simulink model "backstepping"  (R2025b)
settings: Solver=VariableStepAuto  StartTime=0.0  StopTime=10.0  RelTol=1e-3
settings Model: Creator=Predrag  LastModifiedBy=Predrag

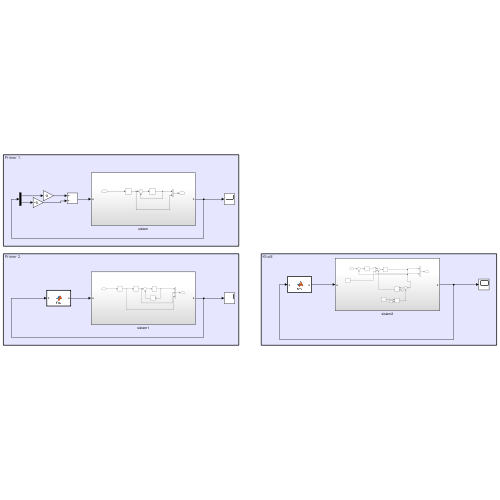
[thumbnail: Simulink's stored preview of the top-level diagram]
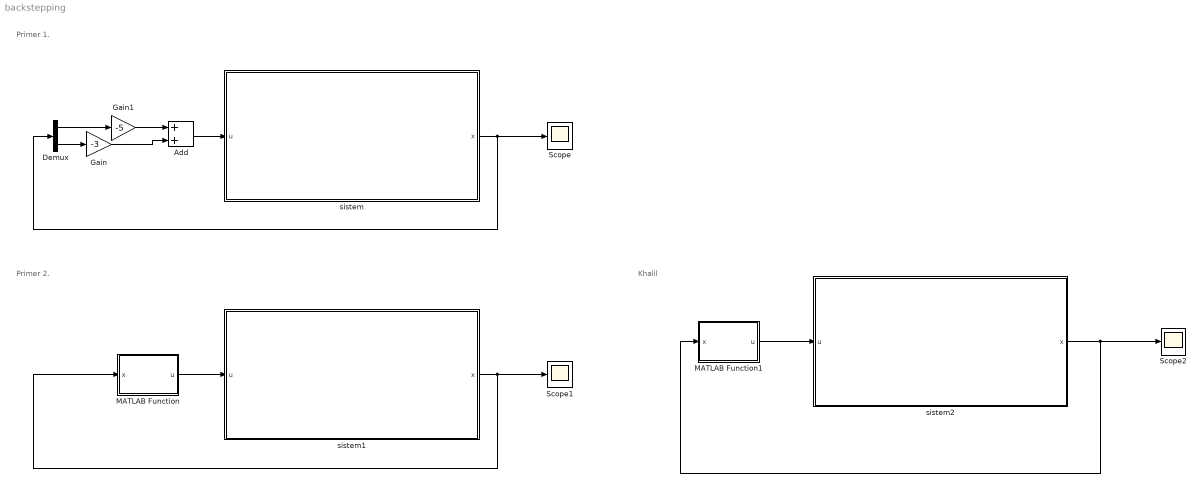
== system backstepping ==
  note: Primer 1.
  note: Primer 2.
  note: Khalil
  Add : Sum
  Demux : Demux  Outputs=2
  Gain : Gain  Gain=-3
  Gain1 : Gain  Gain=-5
  MATLAB Function : MATLAB Function  TreatAsAtomicUnit=on
  MATLAB Function1 : MATLAB Function  TreatAsAtomicUnit=on
  Scope : Scope
      settings: ActiveDisplayYMinimum=-1  ActiveDisplayYMaximum=1
  Scope1 : Scope
      settings: ActiveDisplayYMinimum=-1  ActiveDisplayYMaximum=1
  Scope2 : Scope
      settings: ActiveDisplayYMinimum=-19.86395048104756  ActiveDisplayYMaximum=178.77555432942808  DataLoggingVariableName=ScopeData2
  sistem : Subsystem
  sistem1 : Subsystem
  sistem2 : Subsystem
  wires:
  sistem/1(x) -> Scope/1, Demux/1
  Demux/1 -> Gain1/1
  Demux/2 -> Gain/1
  Gain1/1 -> Add/1
  Gain/1 -> Add/2
  Add/1 -> sistem/1(u)
  sistem1/1(x) -> MATLAB Function/1(x), Scope1/1
  MATLAB Function/1(u) -> sistem1/1(u)
  MATLAB Function1/1(u) -> sistem2/1(u)
  sistem2/1(x) -> MATLAB Function1/1(x), Scope2/1

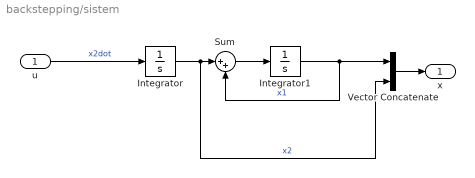
== system backstepping/sistem ==
  u : Inport
  Integrator : Integrator  InitialCondition=1
  Integrator1 : Integrator  InitialCondition=1
  Sum : Sum  Inputs=|++
  Vector Concatenate : Concatenate
  x : Outport
  wires:
  u/1 -> Integrator/1  "x2dot"
  Integrator1/1 -> Vector Concatenate/1, Sum/2  "x1"
  Integrator/1 -> Vector Concatenate/2, Sum/1  "x2"
  Sum/1 -> Integrator1/1
  Vector Concatenate/1 -> x/1

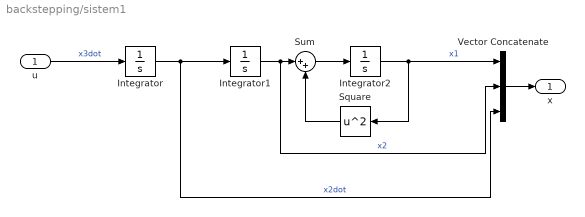
== system backstepping/sistem1 ==
  u : Inport
  Integrator : Integrator  InitialCondition=1
  Integrator1 : Integrator
  Integrator2 : Integrator
  Square : Math  Operator=square
  Sum : Sum  Inputs=|++
  Vector Concatenate : Concatenate  NumInputs=3
  x : Outport
  wires:
  Vector Concatenate/1 -> x/1
  u/1 -> Integrator/1  "x3dot"
  Integrator/1 -> Vector Concatenate/3, Integrator1/1  "x2dot"
  Integrator1/1 -> Vector Concatenate/2, Sum/1  "x2"
  Sum/1 -> Integrator2/1
  Integrator2/1 -> Square/1, Vector Concatenate/1  "x1"
  Square/1 -> Sum/2

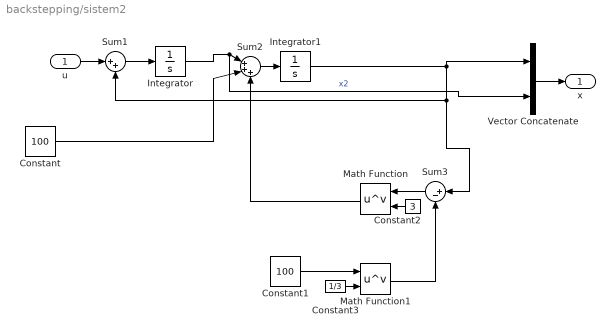
== system backstepping/sistem2 ==
  u : Inport
  Constant : Constant  Value=100
  Constant1 : Constant  Value=100
  Constant2 : Constant  Value=3
  Constant3 : Constant  Value=1/3
  Integrator : Integrator
  Integrator1 : Integrator
  Math Function : Math  Operator=pow
  Math Function1 : Math  Operator=pow
  Sum1 : Sum  Inputs=|++
  Sum2 : Sum  Inputs=|+++
  Sum3 : Sum  Inputs=|+-
  Vector Concatenate : Concatenate
  x : Outport
  wires:
  Integrator1/1 -> Vector Concatenate/1, Sum3/1, Sum1/2
  Vector Concatenate/1 -> x/1
  u/1 -> Sum1/1
  Sum1/1 -> Integrator/1
  Integrator/1 -> Vector Concatenate/2, Sum2/1  "x2"
  Sum2/1 -> Integrator1/1
  Constant/1 -> Sum2/2
  Sum3/1 -> Math Function/1
  Constant2/1 -> Math Function/2
  Constant3/1 -> Math Function1/2
  Constant1/1 -> Math Function1/1
  Math Function1/1 -> Sum3/2
  Math Function/1 -> Sum2/3

== matlab function backstepping/MATLAB Function ==
  data: x input; u output
function u = fcn(x)

x1 = x(1, 1);
x2 = x(2, 1);
x3 = x(3, 1);


a = 1;
l = 1;
g = 1;

v2 = -(1 + a * l)*x1 - (a+ l) * x1^2 - 2*x1^3 - (a + l)*x2 - 2*x1*x2;
z3 = x3 - v2;

dphi2 = (- (1 + a*l) -2*x2 - (2*(a+l)*x1 + 6*x1^2)*(x1^2 + x2))*(x1^2 + x2) - ((a+l) + 2*x1)*x3;

u = -g * z3 + dphi2;

== matlab function backstepping/MATLAB Function1 ==
  data: x input; u output
function u = fcn(x)

x1 = x(1, 1);
x2 = x(2, 1);

a = 100;
phi = -a - (x1 - a^(1/3))^3 - x1;

u = 3 *(x1 - a^(1/3))^2 * (x2 - x1 - phi) - 3*x1;
